simulink model "iksolvermodel_limited"  (R2025b)
settings: Solver=ode4  StartTime=0.0  StopTime=10  FixedStep=0.02  RelTol=1e-3
values from neighbouring files (symbols this model uses):
  joint_angles = [0, 0.8, -1.2, 0.9, 0] - joint_offsets    [fk_visual.m]
  joint_offsets = [2.94961, 2.70526, -2.54818, 3.36174, 2.92343]    [fk_visual.m]
settings Model: Creator=sinan  LastModifiedBy=sinanair

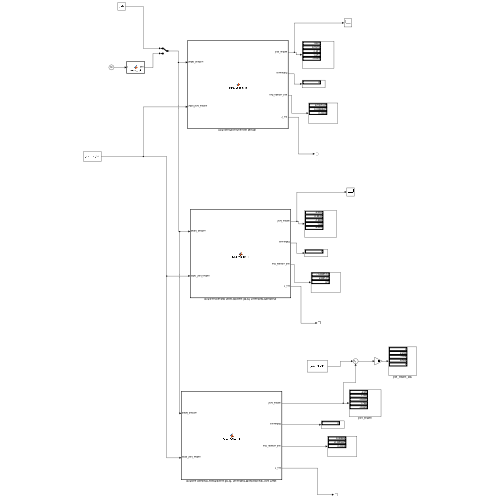
[thumbnail: Simulink's stored preview of the top-level diagram]
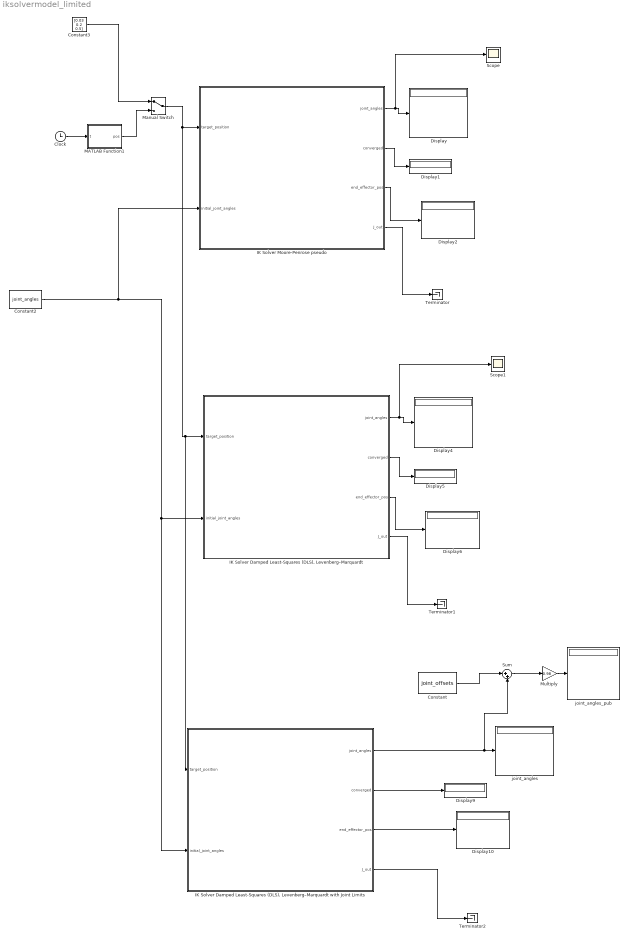
== system iksolvermodel_limited ==
  Clock : Clock
  Constant : Constant  Value=joint_offsets
  Constant2 : Constant  Value=joint_angles
  Constant3 : Constant  Value=[0.03 0.2 0.5]
  Display{,1..2,4..6,9..10} (8 alike) : Display
  "IK Solver Damped Least-Squares (DLS), Levenberg–Marquardt" : MATLAB Function  TreatAsAtomicUnit=on
  "IK Solver Damped Least-Squares (DLS), Levenberg–Marquardt with Joint Limits" : MATLAB Function  TreatAsAtomicUnit=on
  "IK Solver Moore-Penrose pseudo " : MATLAB Function  TreatAsAtomicUnit=on
  MATLAB Function1 : MATLAB Function  TreatAsAtomicUnit=on
  Manual Switch : ManualSwitch
  Multiply : Gain  Gain=0.98
  Scope : Scope
      settings: ActiveDisplayYMinimum=-2.56262  ActiveDisplayYMaximum=4.32205
  Scope1 : Scope
      settings: ActiveDisplayYMinimum=-2.5514  ActiveDisplayYMaximum=4.32106
  Sum : Sum  Inputs=|++
  Terminator : Terminator
  Terminator1 : Terminator
  Terminator2 : Terminator
  joint_angles : Display
  joint_angles_pub : Display
  wires:
  Constant2/1 -> "IK Solver Moore-Penrose pseudo "/2(initial_joint_angles), "IK Solver Damped Least-Squares (DLS), Levenberg–Marquardt with Joint Limits"/2(initial_joint_angles), "IK Solver Damped Least-Squares (DLS), Levenberg–Marquardt"/2(initial_joint_angles)
  "IK Solver Moore-Penrose pseudo "/1(joint_angles) -> Scope/1, Display/1
  "IK Solver Moore-Penrose pseudo "/2(converged) -> Display1/1
  "IK Solver Moore-Penrose pseudo "/3(end_effector_pos) -> Display2/1
  "IK Solver Moore-Penrose pseudo "/4(J_out) -> Terminator/1
  Clock/1 -> MATLAB Function1/1(t)
  "IK Solver Damped Least-Squares (DLS), Levenberg–Marquardt"/4(J_out) -> Terminator1/1
  "IK Solver Damped Least-Squares (DLS), Levenberg–Marquardt"/3(end_effector_pos) -> Display6/1
  "IK Solver Damped Least-Squares (DLS), Levenberg–Marquardt"/2(converged) -> Display5/1
  "IK Solver Damped Least-Squares (DLS), Levenberg–Marquardt"/1(joint_angles) -> Display4/1, Scope1/1
  "IK Solver Damped Least-Squares (DLS), Levenberg–Marquardt with Joint Limits"/3(end_effector_pos) -> Display10/1
  "IK Solver Damped Least-Squares (DLS), Levenberg–Marquardt with Joint Limits"/2(converged) -> Display9/1
  "IK Solver Damped Least-Squares (DLS), Levenberg–Marquardt with Joint Limits"/4(J_out) -> Terminator2/1
  Constant3/1 -> Manual Switch/1
  MATLAB Function1/1(pos) -> Manual Switch/2
  Manual Switch/1 -> "IK Solver Damped Least-Squares (DLS), Levenberg–Marquardt with Joint Limits"/1(target_position), "IK Solver Damped Least-Squares (DLS), Levenberg–Marquardt"/1(target_position), "IK Solver Moore-Penrose pseudo "/1(target_position)
  "IK Solver Damped Least-Squares (DLS), Levenberg–Marquardt with Joint Limits"/1(joint_angles) -> Sum/2, joint_angles/1
  Sum/1 -> Multiply/1
  Constant/1 -> Sum/1
  Multiply/1 -> joint_angles_pub/1

== matlab function iksolvermodel_limited/MATLAB Function1 ==
  data: t input; pos output
function pos = circle_ref(t)
%#codegen   % Simulink Uygunluğu
R     = 0.10;          % yarıçap [m]
Trev  = 5;             % 1 tur süresi [s]
w     = 2*pi/Trev;     % açısal hız [rad/s]
x0    = 0.323;         % sabit x [m]
z0    = 0.074;         % daire merkezi z [m]

y =  R * cos(w*t);
z =  z0 + R * sin(w*t);
pos = [x0; y; z];      % 3×1 hedef pozisyonu
end

== matlab function iksolvermodel_limited/IK Solver Moore-Penrose pseudo  ==
  data: target_position input; joint_angles output; initial_joint_angles input; converged output; end_effector_pos output; J_out output
function [joint_angles, converged, end_effector_pos, J_out] = kuka_youbot_ik( ...
                                   target_position, initial_joint_angles)
%#codegen   % Simulink / Embedded Coder uyum etiketi

%% Sabitler
MAX_ITER = int32(1000);
EPS_POS  = 1e-4;
ALPHA    = 0.10;

%% Başlangıç
joint_angles = initial_joint_angles(:);   % 5×1
converged    = false;
target_p     = target_position(:);        % 3×1

%% İteratif IK
for k = int32(1):MAX_ITER
    T_current = forward_kinematics(joint_angles);
    cur_p     = T_current(1:3,4);
    err       = target_p - cur_p;

    if norm(err) < EPS_POS
        converged = true;
        break;
    end

    J      = compute_jacobian(joint_angles);
    dtheta = ALPHA * pinv(J(1:3,:)) * err;   % yalnızca pozisyonel kısım
    joint_angles = joint_angles + dtheta;
end

%% Nihai çıktılar
T_ee              = forward_kinematics(joint_angles); % 4×4
end_effector_pos  = T_ee(1:3,4);                      % 3×1
J_out             = compute_jacobian(joint_angles);   % 6×5
end   % ===== Ana fonksiyon sonu =====


%% -------------------------------------------------
function T = forward_kinematics(q)
DH =[ 0.033,  pi/2,  0.147,  -q(1);
       0.155,  0,     0,      q(2)+pi/2;
       0.135,  0,     0,      q(3);
       0,      pi/2,  0,      q(4)+pi/2;
       0,      0,     0.187, -q(5) ];
T = eye(4);
for i = 1:5
    T = T * dh_matrix(DH(i,1), DH(i,2), DH(i,3), DH(i,4));
end
end


function J = compute_jacobian(q)
DH = [ 0.033,  pi/2,  0.147,  -q(1);
       0.155,  0,     0,      q(2)+pi/2;
       0.135,  0,     0,      q(3);
       0,      pi/2,  0,      q(4)+pi/2;
       0,      0,     0.187, -q(5) ];

T   = eye(4);
Ts  = zeros(4,4,6);                % sabit boyut
Ts(:,:,1) = T;

for i = 1:5
    T = T * dh_matrix(DH(i,1), DH(i,2), DH(i,3), DH(i,4));
    Ts(:,:,i+1) = T;
end

pe = T(1:3,4);
J  = zeros(6,5);

for i = 1:5
    z   = Ts(1:3,3,i);
    p   = Ts(1:3,4,i);
    J(1:3,i) = cross(z, pe - p);   % lineer kısım
    J(4:6,i) = z;                  % açısal kısım
end
end


function T = dh_matrix(a, alpha, d, theta)
T = [cos(theta), -sin(theta)*cos(alpha),  sin(theta)*sin(alpha), a*cos(theta);
     sin(theta),  cos(theta)*cos(alpha), -cos(theta)*sin(alpha), a*sin(theta);
     0,           sin(alpha),             cos(alpha),            d;
     0,           0,                      0,                     1];
end

== matlab function iksolvermodel_limited/IK Solver Damped Least-Squares (DLS), Levenberg–Marquardt ==
  data: target_position input; joint_angles output; initial_joint_angles input; converged output; end_effector_pos output; J_out output
function [joint_angles, converged, end_effector_pos, J_out] = kuka_youbot_ik( ...
                                   target_position, initial_joint_angles)
%#codegen   % Simulink / Embedded Coder uyum etiketi

%% Sabitler
MAX_ITER = int32(1000);
EPS_POS  = 1e-4;
ALPHA    = 0.5;
LAMBDA   = 0.9;   % Damped Least-Squares lambda katsayısı

%% Başlangıç
joint_angles = initial_joint_angles(:);   % 5×1
converged    = false;
target_p     = target_position(:);        % 3×1

%% İteratif IK
for k = int32(1):MAX_ITER
    T_current = forward_kinematics(joint_angles);
    cur_p     = T_current(1:3,4);
    err       = target_p - cur_p;

    if norm(err) < EPS_POS
        converged = true;
        break;
    end

    J      = compute_jacobian(joint_angles);  % 6×5
    Jv     = J(1:3,:);                        % sadece pozisyonel
    H      = Jv' * Jv;
    dtheta = ALPHA * (H + (LAMBDA^2)*eye(5)) \ (Jv' * err);

    joint_angles = joint_angles + dtheta;
end

%% Nihai çıktılar
T_ee              = forward_kinematics(joint_angles); % 4×4
end_effector_pos  = T_ee(1:3,4);                      % 3×1
J_out             = compute_jacobian(joint_angles);   % 6×5
end   % ===== Ana fonksiyon sonu =====


%% -------------------------------------------------
function T = forward_kinematics(q)
DH = [ 0.033,  pi/2,  0.147,  -q(1);
       0.155,  0,     0,      q(2)+pi/2;
       0.135,  0,     0,      q(3);
       0,      pi/2,  0,      q(4)+pi/2;
       0,      0,     0.187, -q(5) ];
T = eye(4);
for i = 1:5
    T = T * dh_matrix(DH(i,1), DH(i,2), DH(i,3), DH(i,4));
end
end


function J = compute_jacobian(q)
DH = [ 0.033,  pi/2,  0.147,  -q(1);
       0.155,  0,     0,      q(2)+pi/2;
       0.135,  0,     0,      q(3);
       0,      pi/2,  0,      q(4)+pi/2;
       0,      0,    0.187, -q(5) ];

T   = eye(4);
Ts  = zeros(4,4,6);
Ts(:,:,1) = T;

for i = 1:5
    T = T * dh_matrix(DH(i,1), DH(i,2), DH(i,3), DH(i,4));
    Ts(:,:,i+1) = T;
end

pe = T(1:3,4);
J  = zeros(6,5);

for i = 1:5
    z        = Ts(1:3,3,i);
    p        = Ts(1:3,4,i);
    J(1:3,i) = cross(z, pe - p);
    J(4:6,i) = z;
end
end


function T = dh_matrix(a, alpha, d, theta)
T = [cos(theta), -sin(theta)*cos(alpha),  sin(theta)*sin(alpha), a*cos(theta);
     sin(theta),  cos(theta)*cos(alpha), -cos(theta)*sin(alpha), a*sin(theta);
     0,           sin(alpha),             cos(alpha),            d;
     0,           0,                      0,                     1];
end

== matlab function iksolvermodel_limited/IK Solver Damped Least-Squares (DLS), Levenberg–Marquardt with Joint Limits ==
  data: target_position input; joint_angles output; initial_joint_angles input; converged output; end_effector_pos output; J_out output
function [joint_angles, converged, end_effector_pos, J_out] = kuka_youbot_ik( ...
                                   target_position, initial_joint_angles)
%#codegen   % Simulink / Embedded Coder uyum etiketi

%% ---- Sabitler
MAX_ITER = int32(1000);
EPS_POS  = 1e-4;
ALPHA    = 0.5;
LAMBDA   = 0.4;   % Damped Least-Squares lambda
STEP_MAX = 0.3;   % Tek iterasyonda izin verilen max |Δθ| (rad)

% Eklem limitleri (rad) [lower, upper]
JOINT_LIMIT_LIST = [ ...
    2.9496, -2.9496;   % arm_joint_1
    -1.1345,  1.5708;   % arm_joint_2
   2.5482,  -2.6354;  % arm_joint_3
    -1.7890, 1.7890;    % arm_joint_4
    2.9234, -2.9234 ];  % arm_joint_5


%% ---- Başlangıç
joint_angles = initial_joint_angles(:);             % 5×1
joint_angles = project_to_limits(joint_angles, JOINT_LIMIT_LIST); % güvenli başla
converged    = false;
target_p     = target_position(:);                  % 3×1

prev_err_norm = inf;

%% ---- İteratif IK
for k = int32(1):MAX_ITER
    T_current = forward_kinematics(joint_angles);
    cur_p     = T_current(1:3,4);
    err       = target_p - cur_p;
    err_norm  = norm(err);

    if err_norm < EPS_POS
        converged = true;
        break;
    end

    % Jacobian (6x5) ve pozisyonel kısmı
    J      = compute_jacobian(joint_angles);
    Jv     = J(1:3,:);

    % ---- Limit farkındalığı: sütun ağırlama
    S   = diag(joint_limit_scales(joint_angles, JOINT_LIMIT_LIST, 0.05)); % [0.05..1]
    Jvs = Jv * S;

    % DLS adımı (sütun ölçeklemeli)
    H      = Jvs' * Jvs;
    rhs    = Jvs' * err;
    dtheta = ALPHA * (H + (LAMBDA^2)*eye(5)) \ rhs;

    % Parametre uzayı ölçeğini geri uygula
    dtheta = S * dtheta;

    % Tek adım sınırı
    dtheta = max(min(dtheta, STEP_MAX), -STEP_MAX);

    % Güncelle ve limit içinde kal
    joint_angles = project_to_limits(joint_angles + dtheta, JOINT_LIMIT_LIST);

    % İlerleme kontrolü
    if err_norm >= prev_err_norm - 1e-9
        ALPHA = 0.5 * ALPHA;
        if ALPHA < 1e-3
            break;
        end
    end
    prev_err_norm = err_norm;
end

%% ---- Nihai çıktılar
T_ee              = forward_kinematics(joint_angles); % 4×4
end_effector_pos  = T_ee(1:3,4);                      % 3×1
J_out             = compute_jacobian(joint_angles);   % 6×5
end   % ===== Ana fonksiyon sonu =====


%% ============================================================
function q_safe = project_to_limits(q, lims)
% Her eklemi [lower, upper] aralığına kırpar
q_safe = min(max(q(:), lims(:,1)), lims(:,2));
end

function s = joint_limit_scales(q, lims, s_floor)
% Limitlere yaklaştıkça azalan ölçek: s_i = 4*r_i*(1-r_i), r∈[0,1]
r = (q(:) - lims(:,1)) ./ max(lims(:,2) - lims(:,1), 1e-9);
r = min(max(r, 0), 1);
s = 4 .* r .* (1 - r);
s = max(s, s_floor);  % aşırı kısılmayı önleyen taban
end

%% -------------------------------------------------
function T = forward_kinematics(q)
% DH parametreleri (offsetsiz)
DH = [ 0.033,  pi/2,  0.147,  -q(1);
       0.155,  0,     0,      q(2)+pi/2;
       0.135,  0,     0,      q(3);
       0,      pi/2,  0,      q(4)+pi/2;
       0,      0,     0.187, -q(5) ];
T = eye(4);
for i = 1:5
    T = T * dh_matrix(DH(i,1), DH(i,2), DH(i,3), DH(i,4));
end
end

function J = compute_jacobian(q)
DH = [ 0.033,  pi/2,  0.147,  -q(1);
       0.155,  0,     0,      q(2)+pi/2;
       0.135,  0,     0,      q(3);
       0,      pi/2,  0,      q(4)+pi/2;
       0,      0,     0.187, -q(5) ];
T   = eye(4);
Ts  = zeros(4,4,6);
Ts(:,:,1) = T;

for i = 1:5
    T = T * dh_matrix(DH(i,1), DH(i,2), DH(i,3), DH(i,4));
    Ts(:,:,i+1) = T;
end

pe = T(1:3,4);
J  = zeros(6,5);

for i = 1:5
    z        = Ts(1:3,3,i);
    p        = Ts(1:3,4,i);
    J(1:3,i) = cross(z, pe - p);
    J(4:6,i) = z;
end
end

function T = dh_matrix(a, alpha, d, theta)
T = [cos(theta), -sin(theta)*cos(alpha),  sin(theta)*sin(alpha), a*cos(theta);
     sin(theta),  cos(theta)*cos(alpha), -cos(theta)*sin(alpha), a*sin(theta);
     0,           sin(alpha),             cos(alpha),            d;
     0,           0,                      0,                     1];
end
